simulink model "ex2"  (R2024b)
settings: Solver=VariableStepAuto  StartTime=0.0  StopTime=10.0  RelTol=1e-3
libraries: simulink x1
settings Model: Creator=matei  LastModifiedBy=matei

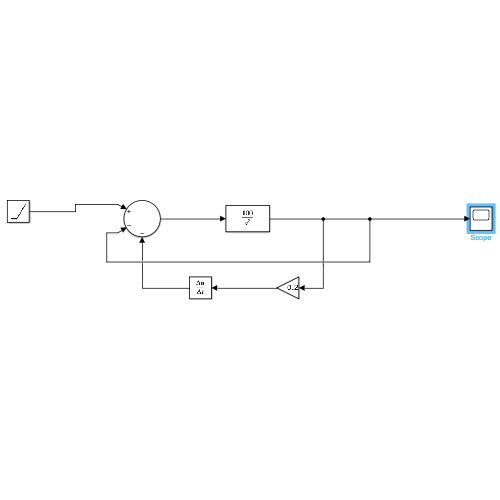
[thumbnail: Simulink's stored preview of the top-level diagram]
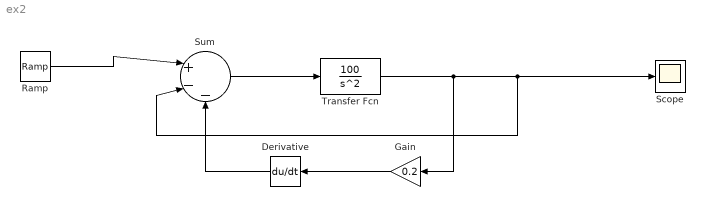
== system ex2 ==
  Derivative : Derivative
  Gain : Gain  Gain=0.2
  Ramp : simulink/Sources/Ramp  slope=1  start=0  InitialOutput=0
  Scope : Scope
  Sum : Sum  Inputs=|+--
  Transfer Fcn : TransferFcn  Numerator=[100]  Denominator=[1 0 0]
  wires:
  Gain/1 -> Derivative/1
  Transfer Fcn/1 -> Scope/1, Sum/2, Gain/1
  Sum/1 -> Transfer Fcn/1
  Ramp/1 -> Sum/1
  Derivative/1 -> Sum/3
